simulink model "A1_MIM0_DigiTwin_4cm_JG_BM_2017b"  (R2017b)
settings: Solver=VariableStepAuto  StartTime=0.0  StopTime=tsim  RelTol=1e-3
InitFcn:
  | tsim=1000
  | sg=1;
  | Ts=500 %500% deseado 890-->Ts modelo
  | wn=5.8335/Ts; %2ord
  | wp=4/Ts; %np=1.5; 1ord
  | wt1=8*wn
  | wt=3.5*wn
  | wt3=3.49*wn
  | nf=2.5; %[1.2 1.5 1.75 2 2.5]
  | %Tfp=1/(np*wp)
  | Tf= 1/(nf*wn) % f del filtro;
  | nf3=5
  | Tf3= 1/(nf3*wn)
  | Rpc=0.09 % cold side resistor
  | Rph= 0.6 % hot side resistor
  | Tamb=273.15+15 % ambiental temp
  | Tin=273.15+15 % initial temp of mass
  | %TinA= 284.9405 % internal air Inicial temp
  | %TinAis=  294.0300 % initial Temp Mass insolat
  | %Tp1=283  %ideal temp of  peltier cells
  | %Tp2=Tp1
  | 
  | %Peltier Cells parameter
  | Th=323 % [K]
  | TinH=298
  | TinC=298 %
  | dTmax=75 % 70.5 [K]
  | Vmax= 16.4 % 13.9 [v]
  | Imax= 6.4 % 4  [A]
  | Rth= (dTmax/(Vmax*Imax))*(2*Th/(Th-dTmax)) % Termal Res [K/W]
  | am= Vmax/ Th %  0.054 Seebeck Coef []
  | ReC=Vmax*(Th-dTmax)/(Th*Imax) %range [1.6 1.96 2.5]
  | %Re= 2.3 %2.65   [2.6584  2.9592 3.26]  at 300 K
  | Mc=0.0135; %0.0045  Cool mass [kg]
  | Mh=0.0135; %0.0045
  | Cesp=1262  %1262.2 345
  | %TinL=300
  | %CespL=100 %45
  | %Mload=100%100-0.065 0.001
  | %Rload=1%5.5
  | 
  | 
  | % --Copper & aluminum plate
  | Da= 8960; %2700 [Kg/m^3] density
  | Qs= 390; %970 Specific heat [J/(Kg*K)]
  | Thi =0.00508; % 0.0033 Thickness [m]
  | L = 0.04; %0.03 length [m]
  | L1=0.035;
  | W=0.04; % 0.03 width  [m]
  | W1=0.01; W2=0.03;  W3=0.015;
  | Va= L*W*Thi % 2,97 E-6 [m^3] Dif of Volume
  | M=Da*Va % 0.00801 [kg]  % Al Dif of Mass
  | 
  | %--- Air Properties
  | Thi_air=0.015 % Thickness of air
  | Dair=1.29 % [Kg/m^3] density
  | Vair= L*W*Thi_air % E-6 [m^3] Dif of Volume
  | Mair=Dair*Vair %  [kg]  % Al Dif of Mass
  | 
  | % thermal conductivity [W/(m*K)]
  | ... (+57 lines)
undefined symbols (not defined in the file or in its folder): TinA, TinAis, ymax, ymin
libraries: fl_lib x233, nesl_utility x61, simulink x6, ee_lib x4
(part 2 of 2)

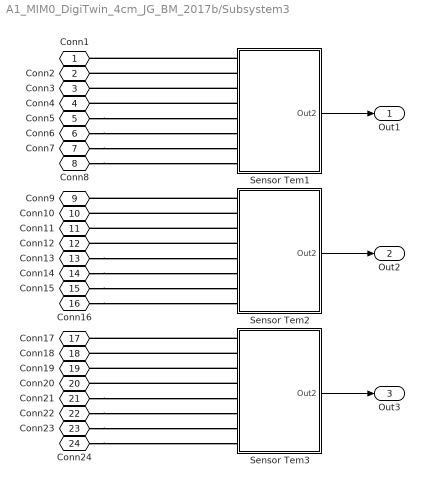
== system A1_MIM0_DigiTwin_4cm_JG_BM_2017b/Subsystem3 ==
  Sensor Tem1 : Subsystem
  Sensor Tem2 : Subsystem
  Sensor Tem3 : Subsystem
  Conn1 : PMIOPort  Side=Left
  Conn2 : PMIOPort  Port=2  Side=Left
  Conn3 : PMIOPort  Port=3  Side=Left
  Conn4 : PMIOPort  Port=4  Side=Left
  Conn5 : PMIOPort  Port=5  Side=Left
  Conn6 : PMIOPort  Port=6  Side=Left
  Conn7 : PMIOPort  Port=7  Side=Left
  Conn8 : PMIOPort  Port=8  Side=Left
  Conn9 : PMIOPort  Port=9  Side=Left
  Conn10 : PMIOPort  Port=10  Side=Left
  Conn11 : PMIOPort  Port=11  Side=Left
  Conn12 : PMIOPort  Port=12  Side=Left
  Conn13 : PMIOPort  Port=13  Side=Left
  Conn14 : PMIOPort  Port=14  Side=Left
  Conn15 : PMIOPort  Port=15  Side=Left
  Conn16 : PMIOPort  Port=16  Side=Left
  Conn17 : PMIOPort  Port=17  Side=Left
  Conn18 : PMIOPort  Port=18  Side=Left
  Conn19 : PMIOPort  Port=19  Side=Left
  Conn20 : PMIOPort  Port=20  Side=Left
  Conn21 : PMIOPort  Port=21  Side=Left
  Conn22 : PMIOPort  Port=22  Side=Left
  Conn23 : PMIOPort  Port=23  Side=Left
  Conn24 : PMIOPort  Port=24  Side=Left
  Out1 : Outport  VectorParamsAs1DForOutWhenUnconnected=off
  Out2 : Outport  Port=2  VectorParamsAs1DForOutWhenUnconnected=off
  Out3 : Outport  Port=3  VectorParamsAs1DForOutWhenUnconnected=off
  wires:
  Sensor Tem1/1(Out2) -> Out1/1
  Sensor Tem2/1(Out2) -> Out2/1
  Sensor Tem3/1(Out2) -> Out3/1
  connections:
  Sensor Tem1/LConn3 -- Conn3/RConn1
  Conn6/RConn1 -- Sensor Tem1/LConn6
  Conn7/RConn1 -- Sensor Tem1/LConn7
  Conn8/RConn1 -- Sensor Tem1/LConn8
  Sensor Tem1/LConn2 -- Conn2/RConn1
  Sensor Tem1/LConn4 -- Conn4/RConn1
  Conn5/RConn1 -- Sensor Tem1/LConn5
  Sensor Tem1/LConn1 -- Conn1/RConn1
  Conn13/RConn1 -- Sensor Tem2/LConn5
  Sensor Tem2/LConn4 -- Conn12/RConn1
  Conn16/RConn1 -- Sensor Tem2/LConn8
  Conn15/RConn1 -- Sensor Tem2/LConn7
  Sensor Tem2/LConn3 -- Conn11/RConn1
  Conn14/RConn1 -- Sensor Tem2/LConn6
  Sensor Tem2/LConn2 -- Conn10/RConn1
  Sensor Tem2/LConn1 -- Conn9/RConn1
  Conn21/RConn1 -- Sensor Tem3/LConn5
  Sensor Tem3/LConn4 -- Conn20/RConn1
  Conn24/RConn1 -- Sensor Tem3/LConn8
  Conn23/RConn1 -- Sensor Tem3/LConn7
  Conn22/RConn1 -- Sensor Tem3/LConn6
  Sensor Tem3/LConn3 -- Conn19/RConn1
  Sensor Tem3/LConn2 -- Conn18/RConn1
  Sensor Tem3/LConn1 -- Conn17/RConn1

== system A1_MIM0_DigiTwin_4cm_JG_BM_2017b/Subsystem4 ==
  PS-Simulink Converter1 : nesl_utility/PS-Simulink Converter  PhysicalDomain=network_engine_domain  SubClassName=ps_output  LeftPortType=input  RightPortType=output  PseudoPeriodic=off  Frequencies=[]  VectorFormat=1-D array  Unit=1  AffineConversion=off
  Temperature Sensor2 : fl_lib/Thermal/Thermal Sensors/Temperature Sensor
  Thermal Reference1 : fl_lib/Thermal/Thermal Elements/Thermal Reference
  Conn1 : PMIOPort  Side=Left
  Out1 : Outport  VectorParamsAs1DForOutWhenUnconnected=off
  wires:
  PS-Simulink Converter1/1 -> Out1/1
  connections:
  Thermal Reference1/LConn1 -- Temperature Sensor2/RConn1
  Temperature Sensor2/LConn1 -- Conn1/RConn1
  Temperature Sensor2/RConn2 -- PS-Simulink Converter1/LConn1

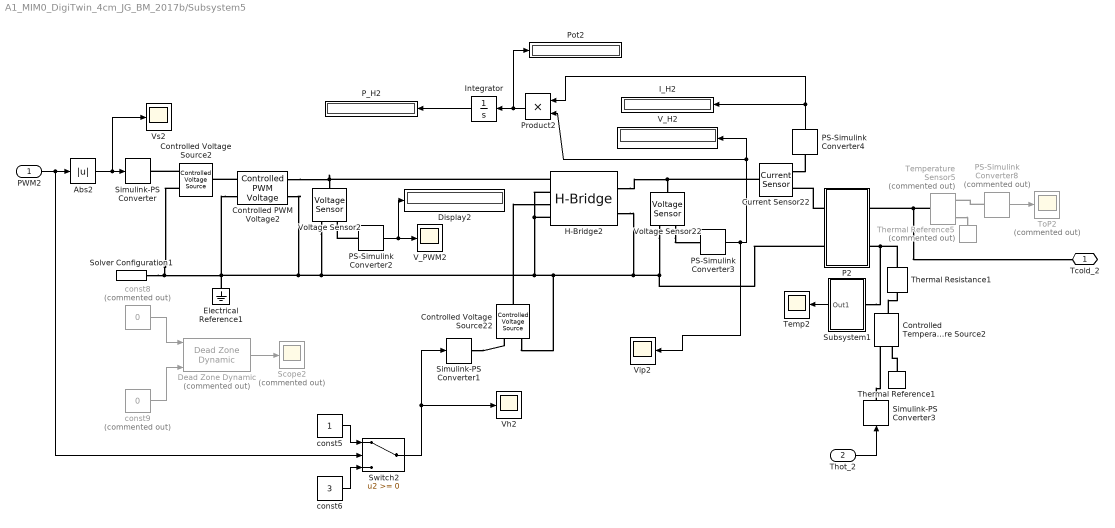
== system A1_MIM0_DigiTwin_4cm_JG_BM_2017b/Subsystem5 ==
  PWM2 : Inport
  Thot_2 : Inport  Port=2
  Abs2 : Abs
  Controlled Temperature Source2 : fl_lib/Thermal/Thermal Sources/Controlled Temperature Source
  Controlled PWM Voltage2 : ee_lib/Integrated Circuits/Controlled PWM Voltage  F=4000 Hz  TD=0 s  pulse_width_offset=0 s  pulse_min=0 s  pwm_or_av=2  event_type=1  sample_time=1e-6 s  Vmin=0 V  Vmax=5 V  Vm=5 V  u_min=0  u_max=1
  Controlled Voltage Source2 : fl_lib/Electrical/Electrical Sources/Controlled Voltage Source
  Controlled Voltage Source22 : fl_lib/Electrical/Electrical Sources/Controlled Voltage Source
  Current Sensor22 : fl_lib/Electrical/Electrical Sensors/Current Sensor
  Dead Zone Dynamic : simulink/Discontinuities/Dead Zone Dynamic  Commented=on
  Display2 : Display
  Electrical Reference1 : fl_lib/Electrical/Electrical Elements/Electrical Reference
  H-Bridge2 : ee_lib/Semiconductors & Converters/Converters/H-Bridge  supply_ports=ee.enum.supply_ports.hidesupply  pwm_or_av=2  regenerative_braking_mode=2  discontinuous=0  freewheeling_mode=1  Rload=10 Ohm  Lload=1e-5 H  F=10 kHz  Venable=2.5 V  Vmax=5.0 V  Vreverse=2.5 V  Vbrake=2.5 V  Vm=12 V  Ron=0.1 Ohm  Don=0.05 Ohm  Goff=1e-6 S  Tmeas=298.15 K  Ron2=0.1 Ohm  Don2=0.05 Ohm  Tmeas2=398.15 K  thermal_mass=100 J/K  initial_temperature=298.15 K
  I_H2 : Display
  Integrator : Integrator
  P2 : Subsystem
  PS-Simulink Converter2 : nesl_utility/PS-Simulink Converter  PhysicalDomain=network_engine_domain  SubClassName=ps_output  LeftPortType=input  RightPortType=output  PseudoPeriodic=off  Frequencies=[]  VectorFormat=1-D array  Unit=1  AffineConversion=off
  PS-Simulink Converter3 : nesl_utility/PS-Simulink Converter  PhysicalDomain=network_engine_domain  SubClassName=ps_output  LeftPortType=input  RightPortType=output  PseudoPeriodic=off  Frequencies=[]  VectorFormat=1-D array  Unit=1  AffineConversion=off
  PS-Simulink Converter4 : nesl_utility/PS-Simulink Converter  PhysicalDomain=network_engine_domain  SubClassName=ps_output  LeftPortType=input  RightPortType=output  PseudoPeriodic=off  Frequencies=[]  VectorFormat=1-D array  Unit=1  AffineConversion=off
  PS-Simulink Converter8 : nesl_utility/PS-Simulink Converter  Commented=on  PhysicalDomain=network_engine_domain  SubClassName=ps_output  LeftPortType=input  RightPortType=output  PseudoPeriodic=off  Frequencies=[]  VectorFormat=1-D array  Unit=1  AffineConversion=off
  P_H2 : Display
  Pot2 : Display
  Product2 : Product  RndMeth=Zero
  Scope2 : Scope  Commented=on
  Simulink-PS Converter : nesl_utility/Simulink-PS Converter  PhysicalDomain=network_engine_domain  SubClassName=ps_input  LeftPortType=input  RightPortType=output  PseudoPeriodic=off  Frequencies=[]  NoiseDistribution=none  NoiseParameters=[]  Unit=1  AffineConversion=off  FilteringAndDerivatives=provide  SimscapeFilterOrder=1  InputFilterTimeConstant=0.001  UdotUserProvided=0
  Simulink-PS Converter1 : nesl_utility/Simulink-PS Converter  PhysicalDomain=network_engine_domain  SubClassName=ps_input  LeftPortType=input  RightPortType=output  PseudoPeriodic=off  Frequencies=[]  NoiseDistribution=none  NoiseParameters=[]  Unit=1  AffineConversion=off  FilteringAndDerivatives=provide  SimscapeFilterOrder=1  InputFilterTimeConstant=0.001  UdotUserProvided=0
  Simulink-PS Converter3 : nesl_utility/Simulink-PS Converter  PhysicalDomain=network_engine_domain  SubClassName=ps_input  LeftPortType=input  RightPortType=output  PseudoPeriodic=off  Frequencies=[]  NoiseDistribution=none  NoiseParameters=[]  Unit=1  AffineConversion=off  FilteringAndDerivatives=provide  SimscapeFilterOrder=1  InputFilterTimeConstant=0.001  UdotUserProvided=0
  Solver Configuration1 : nesl_utility/Solver Configuration  PhysicalDomain=network_engine_domain  SubClassName=solver  LeftPortType=input  RightPortType=generic  Tones=[]  Harmonics=[]  SimulateNoise=off  Profile=off  UseLocalSampling=off  EnableSwitchedLinearOptims=on  FrequencyDomain=off  UseCCode=off  RelTol=0.001  AbsTol=1e-06  MinStep=1e-09  ToWorkspace=off  RevertToSquareIcSolve=off  NumHomotopyIterations=100  PhasorMode=off  PhasorModeNumHarmonics=1  ConsistencySolver=NEWTON_FTOL  IndexReductionMethod=DerivativeReplacement  DoDC=off  ResidualTolerance=1e-09  ConsistencyTolSource=GLOBAL  ConsistencyAbsTol=0.001  ConsistencyRelTol=0.001  ConsistencyTolFactor=0.001  UseLocalSolver=off  LocalSolverChoice=NE_BACKWARD_EULER_ADVANCER  ResolveIndetEquations=on  FunctionEvalNumThread=1  LocalSolverSampleTime=0.001  DoFixedCost=off  MaxNonlinIter=3  MaxModeIter=2  ComputeImpulses=off  ImpulseIterations=2  LinearAlgebra=Sparse  LinearAlgebraNumThread=0  EquationFormulation=NE_TIME_EF  DelaysMemoryBudget=1024  AutomaticFiltering=on  FilteringTimeConstant=0.001  PartitionStorageMethod=AS_NEEDED  PartitionMemoryBudget=1024  PartitionMethod=FAST
  Subsystem1 : Subsystem
  Switch2 : Switch
  Temp2 : Scope
  Temperature Sensor5 : fl_lib/Thermal/Thermal Sensors/Temperature Sensor  Commented=on
  Thermal Reference1 : fl_lib/Thermal/Thermal Elements/Thermal Reference
  Thermal Reference5 : fl_lib/Thermal/Thermal Elements/Thermal Reference  Commented=on
  Thermal Resistance1 : fl_lib/Thermal/Thermal Elements/Thermal Resistance  resistance=Rph K/W  T_specify=off  T_priority=None  T=0 K  T_nominal_specify=off  T_nominal_unit=K  T_nominal_value=1  Q_specify=off  Q_priority=None  Q=0 W  Q_nominal_specify=off  Q_nominal_unit=W  Q_nominal_value=1
  ToP2 : Scope  Commented=on
  V_H2 : Display
  V_PWM2 : Scope
  Vh2 : Scope
  Vip2 : Scope
  Voltage Sensor2 : fl_lib/Electrical/Electrical Sensors/Voltage Sensor
  Voltage Sensor22 : fl_lib/Electrical/Electrical Sensors/Voltage Sensor
  Vs2 : Scope
  const5 : Constant
  const6 : Constant  Value=3
  const8 : Constant  Commented=on  Value=0
  const9 : Constant  Commented=on  Value=0
  Tcold_2 : PMIOPort  Side=Right
  wires:
  const8/1 -> Dead Zone Dynamic/1
  Dead Zone Dynamic/1 -> Scope2/1
  const9/1 -> Dead Zone Dynamic/3
  Product2/1 -> Integrator/1, Pot2/1
  PS-Simulink Converter3/1 -> V_H2/1, Product2/2, Vip2/1
  PS-Simulink Converter4/1 -> I_H2/1, Product2/1
  Integrator/1 -> P_H2/1
  Abs2/1 -> Simulink-PS Converter/1, Vs2/1
  const6/1 -> Switch2/3
  PWM2/1 -> Abs2/1, Switch2/2
  const5/1 -> Switch2/1
  Thot_2/1 -> Simulink-PS Converter3/1
  Subsystem1/1(Out1) -> Temp2/1
  PS-Simulink Converter2/1 -> V_PWM2/1, Display2/1
  PS-Simulink Converter8/1 -> ToP2/1
  Switch2/1 -> Vh2/1, Simulink-PS Converter1/1
  connections:
  Controlled PWM Voltage2/LConn2 -- Controlled PWM Voltage2/RConn2 -- Voltage Sensor2/RConn2 -- H-Bridge2/RConn2 -- Voltage Sensor22/RConn2 -- P2/LConn2 -- Controlled Voltage Source22/RConn2 -- H-Bridge2/LConn2 -- H-Bridge2/LConn4 -- Solver Configuration1/RConn1 -- Controlled Voltage Source2/RConn2 -- Electrical Reference1/LConn1
  Controlled Temperature Source2/LConn1 -- Thermal Resistance1/LConn1
  Thermal Reference1/LConn1 -- Controlled Temperature Source2/RConn2
  Simulink-PS Converter3/RConn1 -- Controlled Temperature Source2/RConn1
  P2/RConn2 -- Subsystem1/LConn1 -- Thermal Resistance1/RConn1
  Current Sensor22/RConn1 -- PS-Simulink Converter4/LConn1
  Voltage Sensor22/LConn1 -- Current Sensor22/LConn1 -- H-Bridge2/RConn1
  PS-Simulink Converter2/LConn1 -- Voltage Sensor2/RConn1
  P2/RConn1 -- Tcold_2/RConn1 -- Temperature Sensor5/LConn1
  Controlled Voltage Source2/RConn1 -- Simulink-PS Converter/RConn1
  Voltage Sensor2/LConn1 -- H-Bridge2/LConn1 -- Controlled PWM Voltage2/RConn1
  Voltage Sensor22/RConn1 -- PS-Simulink Converter3/LConn1
  PS-Simulink Converter8/LConn1 -- Temperature Sensor5/RConn2
  Controlled Voltage Source22/LConn1 -- H-Bridge2/LConn3
  Controlled PWM Voltage2/LConn1 -- Controlled Voltage Source2/LConn1
  P2/LConn1 -- Current Sensor22/RConn2
  Simulink-PS Converter1/RConn1 -- Controlled Voltage Source22/RConn1
  Temperature Sensor5/RConn1 -- Thermal Reference5/LConn1

== system A1_MIM0_DigiTwin_4cm_JG_BM_2017b/Subsystem6 ==
  PS-Simulink Converter1 : nesl_utility/PS-Simulink Converter  PhysicalDomain=network_engine_domain  SubClassName=ps_output  LeftPortType=input  RightPortType=output  PseudoPeriodic=off  Frequencies=[]  VectorFormat=1-D array  Unit=1  AffineConversion=off
  Temperature Sensor2 : fl_lib/Thermal/Thermal Sensors/Temperature Sensor
  Thermal Reference1 : fl_lib/Thermal/Thermal Elements/Thermal Reference
  Conn1 : PMIOPort  Side=Left
  Out1 : Outport  VectorParamsAs1DForOutWhenUnconnected=off
  wires:
  PS-Simulink Converter1/1 -> Out1/1
  connections:
  Temperature Sensor2/RConn2 -- PS-Simulink Converter1/LConn1
  Temperature Sensor2/LConn1 -- Conn1/RConn1
  Thermal Reference1/LConn1 -- Temperature Sensor2/RConn1

== system A1_MIM0_DigiTwin_4cm_JG_BM_2017b/Subsystem7 ==
  PS-Simulink Converter1 : nesl_utility/PS-Simulink Converter  PhysicalDomain=network_engine_domain  SubClassName=ps_output  LeftPortType=input  RightPortType=output  PseudoPeriodic=off  Frequencies=[]  VectorFormat=1-D array  Unit=1  AffineConversion=off
  Temperature Sensor2 : fl_lib/Thermal/Thermal Sensors/Temperature Sensor
  Thermal Reference4 : fl_lib/Thermal/Thermal Elements/Thermal Reference
  Conn1 : PMIOPort  Side=Left
  Out1 : Outport  VectorParamsAs1DForOutWhenUnconnected=off
  wires:
  PS-Simulink Converter1/1 -> Out1/1
  connections:
  Thermal Reference4/LConn1 -- Temperature Sensor2/RConn1
  PS-Simulink Converter1/LConn1 -- Temperature Sensor2/RConn2
  Temperature Sensor2/LConn1 -- Conn1/RConn1

== system A1_MIM0_DigiTwin_4cm_JG_BM_2017b/Ts_98%1 ==
  note: Subsystem
  note: Subsystem1
  In1 : Inport
  Constant1 : Constant  Commented=on  Value=ymax
  Constant4 : Constant  Value=298
  Constant5 : Constant  Commented=on  Value=ymin
  Manual Switch : ManualSwitch  Commented=on  CurrentSetting=0
  MpSinF : TransferFcn  Numerator=1  Denominator=[(1/wp) 1]
  MrF1ord1 : TransferFcn  Numerator=[wn^2*Tf wn^2]  Denominator=[1 2*wn*sg wn^2 ]
  MrWn1 : TransferFcn  Numerator=[wn^2]  Denominator=[1 2*wn*sg wn^2 ]
  Product : Product
  Product1 : Product
  Repeating Sequence Stair1 : simulink/Sources/Repeating Sequence Stair  OutValues=[ 0 1 0 ]'  tsamp=2000  OutMin=[]  OutMax=[]  OutDataTypeStr=float('double')  OutputDataTypeScalingMode=Specify via dialog  OutDataType=float('double')  ConRadixGroup=Best Precision: Vector-wise  OutScaling=2^-12
  Repeating Sequence Stair2 : simulink/Sources/Repeating Sequence Stair  OutValues=[ 1 0 1 ]'  tsamp=2000  OutMin=[]  OutMax=[]  OutDataTypeStr=float('double')  OutputDataTypeScalingMode=Specify via dialog  OutDataType=float('double')  ConRadixGroup=Best Precision: Vector-wise  OutScaling=2^-12
  Subtract : Sum  Inputs=+-
  Subtract1 : Sum
  Yab : Constant  Value=-10.2170e+000
  Ymax : Constant  Value=44.2455e+000
  Ymin : Constant  Value=-11.3285e+000
  yar : Constant  Value=43.3605e+000
  Peltier : Outport  VectorParamsAs1DForOutWhenUnconnected=off
  Out2 : Outport  Port=2  VectorParamsAs1DForOutWhenUnconnected=off
  Out3 : Outport  Port=3  VectorParamsAs1DForOutWhenUnconnected=off
  Ms : Outport  Port=4  VectorParamsAs1DForOutWhenUnconnected=off
  MsFp : Outport  Port=5  VectorParamsAs1DForOutWhenUnconnected=off
  Mp : Outport  Port=6  VectorParamsAs1DForOutWhenUnconnected=off
  wires:
  yar/1 -> Out2/1
  Yab/1 -> Out3/1
  Constant4/1 -> Subtract/2
  Subtract/1 -> Peltier/1
  In1/1 -> Subtract/1
  Product1/1 -> Subtract1/2
  Ymax/1 -> Product/1
  Product/1 -> Subtract1/1
  Repeating Sequence Stair2/1 -> Product/2
  Repeating Sequence Stair1/1 -> Product1/1
  Ymin/1 -> Product1/2
  MrWn1/1 -> Ms/1
  MrF1ord1/1 -> MsFp/1
  MpSinF/1 -> Mp/1
  Subtract1/1 -> MrWn1/1, MpSinF/1, MrF1ord1/1

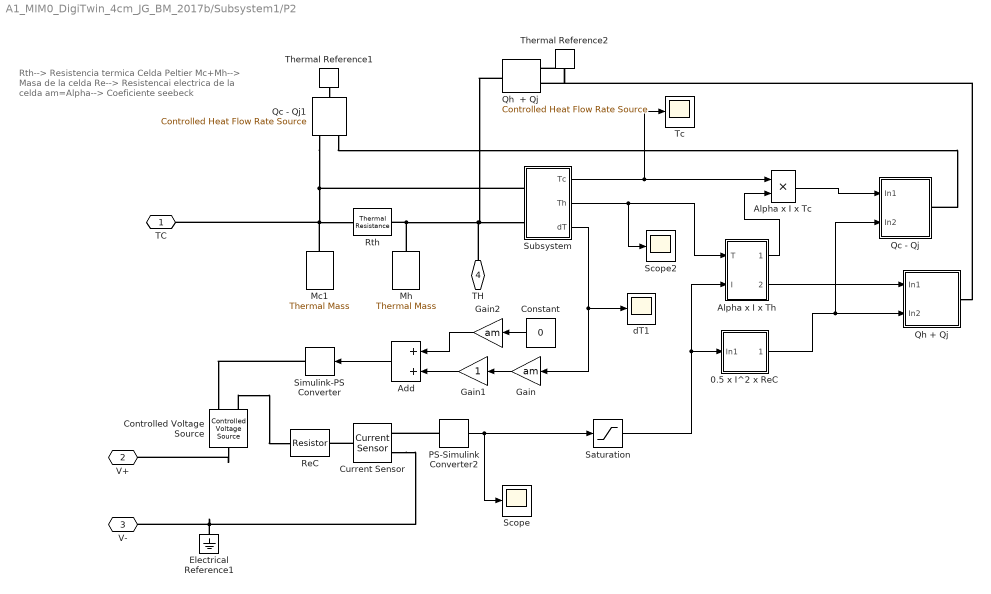
== system A1_MIM0_DigiTwin_4cm_JG_BM_2017b/Subsystem1/P2 ==
  note: Rth-->                  Resistencia termica Celda Peltier
      | Mc+Mh-->            Masa de la celda
      | Re-->                  Resistencai electrica de la celda
      | am=Alpha-->       Coeficiente seebeck
  0.5 x I^2 x ReC : Subsystem
  Add : Sum
  Alpha x I x Tc : Product
  Alpha x I x Th : Subsystem
  Constant : Constant  Value=0
  Controlled Voltage Source : fl_lib/Electrical/Electrical Sources/Controlled Voltage Source
  Current Sensor : fl_lib/Electrical/Electrical Sensors/Current Sensor
  Electrical Reference1 : fl_lib/Electrical/Electrical Elements/Electrical Reference
  Gain : Gain  Gain=am
  Gain1 : Gain
  Gain2 : Gain  Gain=am
  Mc1 : fl_lib/Thermal/Thermal Elements/Thermal Mass  mass=Mc kg  sp_heat=Cesp J/kg/K  num_ports=foundation.enum.numPorts2.one  T_specify=on  T_priority=High  T=TinC K  T_nominal_specify=off  T_nominal_unit=K  T_nominal_value=1  Q_specify=off  Q_priority=None  Q=0 W  Q_nominal_specify=off  Q_nominal_unit=W  Q_nominal_value=1
  Mh : fl_lib/Thermal/Thermal Elements/Thermal Mass  mass=Mh kg  sp_heat=Cesp J/kg/K  num_ports=foundation.enum.numPorts2.one  T_specify=on  T_priority=High  T=TinH K  T_nominal_specify=off  T_nominal_unit=K  T_nominal_value=1  Q_specify=off  Q_priority=None  Q=0 W  Q_nominal_specify=off  Q_nominal_unit=W  Q_nominal_value=1
  PS-Simulink Converter2 : nesl_utility/PS-Simulink Converter  PhysicalDomain=network_engine_domain  SubClassName=ps_output  LeftPortType=input  RightPortType=output  PseudoPeriodic=off  Frequencies=[]  VectorFormat=1-D array  Unit=1  AffineConversion=off
  "Qc - Qj " : Subsystem
  "Qc - Qj1 " : fl_lib/Thermal/Thermal Sources/Controlled Heat Flow Rate Source
  Qh  + Qj : fl_lib/Thermal/Thermal Sources/Controlled Heat Flow Rate Source
  "Qh + Qj " : Subsystem
  ReC : fl_lib/Electrical/Electrical Elements/Resistor  R=ReC Ohm  i_specify=off  i_priority=None  i=0 A  i_nominal_specify=off  i_nominal_unit=A  i_nominal_value=1  v_specify=off  v_priority=None  v=0 V  v_nominal_specify=off  v_nominal_unit=V  v_nominal_value=1
  Rth : fl_lib/Thermal/Thermal Elements/Thermal Resistance  resistance=Rth K/W  T_specify=off  T_priority=None  T=0 K  T_nominal_specify=off  T_nominal_unit=K  T_nominal_value=1  Q_specify=off  Q_priority=None  Q=0 W  Q_nominal_specify=off  Q_nominal_unit=W  Q_nominal_value=1
  Saturation : Saturate  UpperLimit=inf  LowerLimit=-inf
  Scope : Scope
  Scope2 : Scope
  Simulink-PS Converter : nesl_utility/Simulink-PS Converter  PhysicalDomain=network_engine_domain  SubClassName=ps_input  LeftPortType=input  RightPortType=output  PseudoPeriodic=off  Frequencies=[]  NoiseDistribution=none  NoiseParameters=[]  Unit=1  AffineConversion=off  FilteringAndDerivatives=provide  SimscapeFilterOrder=1  InputFilterTimeConstant=0.001  UdotUserProvided=0
  Subsystem : Subsystem
  Tc : Scope
  Thermal Reference1 : fl_lib/Thermal/Thermal Elements/Thermal Reference
  Thermal Reference2 : fl_lib/Thermal/Thermal Elements/Thermal Reference
  dT1 : Scope
  TC : PMIOPort  Side=Right
  V+ : PMIOPort  Port=2  Side=Left
  V- : PMIOPort  Port=3  Side=Left
  TH : PMIOPort  Port=4  Side=Right
  wires:
  PS-Simulink Converter2/1 -> Scope/1, Saturation/1
  0.5 x I^2 x ReC/1(Out1) -> "Qc - Qj "/2(In2), "Qh + Qj "/2(In2)
  Subsystem/1(Tc) -> Tc/1, Alpha x I x Tc/1
  Alpha x I x Th/1(Out1) -> Alpha x I x Tc/2
  Alpha x I x Tc/1 -> "Qc - Qj "/1(In1)
  Alpha x I x Th/2(Out2) -> "Qh + Qj "/1(In1)
  Subsystem/2(Th) -> Scope2/1, Alpha x I x Th/1(T)
  Saturation/1 -> Alpha x I x Th/2(I), 0.5 x I^2 x ReC/1(In1)
  Subsystem/3(dT) -> Gain/1, dT1/1
  Gain/1 -> Gain1/1
  Gain1/1 -> Add/2
  Constant/1 -> Gain2/1
  Add/1 -> Simulink-PS Converter/1
  Gain2/1 -> Add/1
  connections:
  Current Sensor/LConn1 -- ReC/RConn1
  Thermal Reference1/LConn1 -- "Qc - Qj1 "/LConn1
  Thermal Reference2/LConn1 -- Qh  + Qj/RConn2
  Mh/LConn1 -- Rth/RConn1 -- Qh  + Qj/LConn1 -- Subsystem/LConn2 -- TH/RConn1
  Simulink-PS Converter/RConn1 -- Controlled Voltage Source/RConn1
  Controlled Voltage Source/RConn2 -- ReC/LConn1
  PS-Simulink Converter2/LConn1 -- Current Sensor/RConn1
  Controlled Voltage Source/LConn1 -- V+/RConn1
  Current Sensor/RConn2 -- V-/RConn1 -- Electrical Reference1/LConn1
  "Qc - Qj1 "/RConn1 -- "Qc - Qj "/RConn1
  "Qh + Qj "/RConn1 -- Qh  + Qj/RConn1
  "Qc - Qj1 "/RConn2 -- Subsystem/LConn1 -- Mc1/LConn1 -- TC/RConn1 -- Rth/LConn1

== system A1_MIM0_DigiTwin_4cm_JG_BM_2017b/Subsystem1/Subsystem1 ==
  PS-Simulink Converter7 : nesl_utility/PS-Simulink Converter  PhysicalDomain=network_engine_domain  SubClassName=ps_output  LeftPortType=input  RightPortType=output  PseudoPeriodic=off  Frequencies=[]  VectorFormat=1-D array  Unit=1  AffineConversion=off
  Temperature Sensor1 : fl_lib/Thermal/Thermal Sensors/Temperature Sensor
  Thermal Reference2 : fl_lib/Thermal/Thermal Elements/Thermal Reference
  Conn1 : PMIOPort  Side=Left
  Out1 : Outport  VectorParamsAs1DForOutWhenUnconnected=off
  wires:
  PS-Simulink Converter7/1 -> Out1/1
  connections:
  Thermal Reference2/LConn1 -- Temperature Sensor1/RConn1
  PS-Simulink Converter7/LConn1 -- Temperature Sensor1/RConn2
  Temperature Sensor1/LConn1 -- Conn1/RConn1

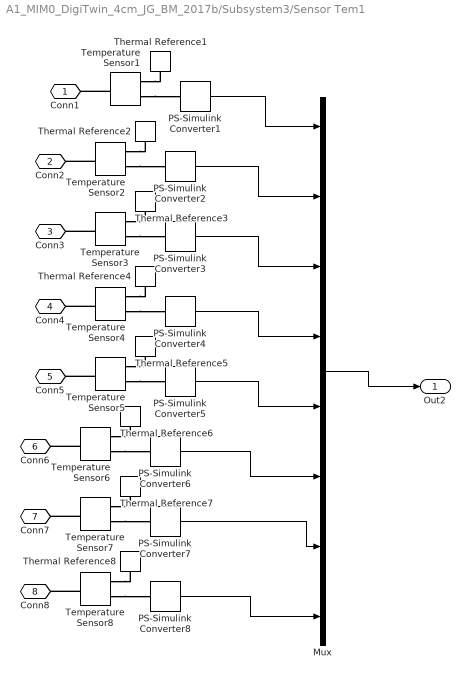
== system A1_MIM0_DigiTwin_4cm_JG_BM_2017b/Subsystem3/Sensor Tem1 ==
  Mux : Mux  Inputs=8
  PS-Simulink Converter{1..8} (8 alike) : nesl_utility/PS-Simulink Converter  PhysicalDomain=network_engine_domain  SubClassName=ps_output  LeftPortType=input  RightPortType=output  PseudoPeriodic=off  Frequencies=[]  VectorFormat=1-D array  Unit=1  AffineConversion=off
  Temperature Sensor{1..8} (8 alike) : fl_lib/Thermal/Thermal Sensors/Temperature Sensor
  Thermal Reference{1..8} (8 alike) : fl_lib/Thermal/Thermal Elements/Thermal Reference
  Conn1 : PMIOPort  Side=Left
  Conn2 : PMIOPort  Port=2  Side=Left
  Conn3 : PMIOPort  Port=3  Side=Left
  Conn4 : PMIOPort  Port=4  Side=Left
  Conn5 : PMIOPort  Port=5  Side=Left
  Conn6 : PMIOPort  Port=6  Side=Left
  Conn7 : PMIOPort  Port=7  Side=Left
  Conn8 : PMIOPort  Port=8  Side=Left
  Out2 : Outport  VectorParamsAs1DForOutWhenUnconnected=off
  wires:
  PS-Simulink Converter5/1 -> Mux/5
  PS-Simulink Converter7/1 -> Mux/7
  PS-Simulink Converter8/1 -> Mux/8
  PS-Simulink Converter6/1 -> Mux/6
  PS-Simulink Converter4/1 -> Mux/4
  PS-Simulink Converter3/1 -> Mux/3
  PS-Simulink Converter1/1 -> Mux/1
  PS-Simulink Converter2/1 -> Mux/2
  Mux/1 -> Out2/1
  connections:
  Temperature Sensor6/RConn2 -- PS-Simulink Converter6/LConn1
  Temperature Sensor5/RConn2 -- PS-Simulink Converter5/LConn1
  Temperature Sensor5/RConn1 -- Thermal Reference5/LConn1
  Temperature Sensor7/RConn2 -- PS-Simulink Converter7/LConn1
  Temperature Sensor6/RConn1 -- Thermal Reference6/LConn1
  Temperature Sensor5/LConn1 -- Conn5/RConn1
  Temperature Sensor6/LConn1 -- Conn6/RConn1
  Temperature Sensor7/LConn1 -- Conn7/RConn1
  Temperature Sensor7/RConn1 -- Thermal Reference7/LConn1
  Temperature Sensor8/RConn1 -- Thermal Reference8/LConn1
  Temperature Sensor8/LConn1 -- Conn8/RConn1
  Temperature Sensor8/RConn2 -- PS-Simulink Converter8/LConn1
  Temperature Sensor4/RConn2 -- PS-Simulink Converter4/LConn1
  Temperature Sensor4/LConn1 -- Conn4/RConn1
  Temperature Sensor4/RConn1 -- Thermal Reference4/LConn1
  Temperature Sensor3/RConn1 -- Thermal Reference3/LConn1
  Temperature Sensor3/LConn1 -- Conn3/RConn1
  Temperature Sensor3/RConn2 -- PS-Simulink Converter3/LConn1
  Temperature Sensor2/RConn1 -- Thermal Reference2/LConn1
  Temperature Sensor2/RConn2 -- PS-Simulink Converter2/LConn1
  Temperature Sensor2/LConn1 -- Conn2/RConn1
  Temperature Sensor1/LConn1 -- Conn1/RConn1
  Temperature Sensor1/RConn2 -- PS-Simulink Converter1/LConn1
  Temperature Sensor1/RConn1 -- Thermal Reference1/LConn1

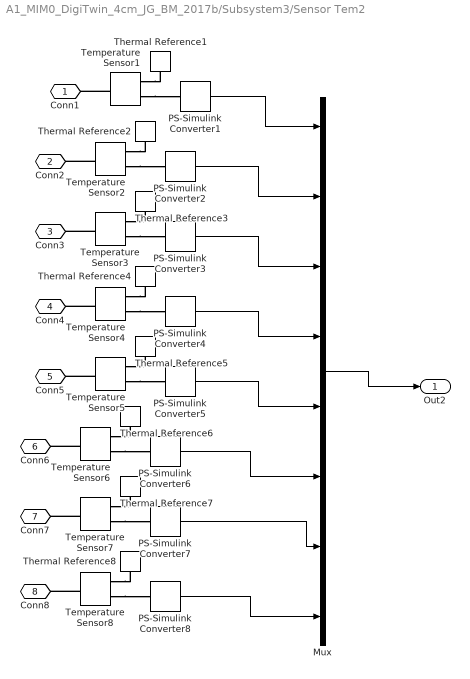
== system A1_MIM0_DigiTwin_4cm_JG_BM_2017b/Subsystem3/Sensor Tem2 ==
  Mux : Mux  Inputs=8
  PS-Simulink Converter{1..8} (8 alike) : nesl_utility/PS-Simulink Converter  PhysicalDomain=network_engine_domain  SubClassName=ps_output  LeftPortType=input  RightPortType=output  PseudoPeriodic=off  Frequencies=[]  VectorFormat=1-D array  Unit=1  AffineConversion=off
  Temperature Sensor{1..8} (8 alike) : fl_lib/Thermal/Thermal Sensors/Temperature Sensor
  Thermal Reference{1..8} (8 alike) : fl_lib/Thermal/Thermal Elements/Thermal Reference
  Conn1 : PMIOPort  Side=Left
  Conn2 : PMIOPort  Port=2  Side=Left
  Conn3 : PMIOPort  Port=3  Side=Left
  Conn4 : PMIOPort  Port=4  Side=Left
  Conn5 : PMIOPort  Port=5  Side=Left
  Conn6 : PMIOPort  Port=6  Side=Left
  Conn7 : PMIOPort  Port=7  Side=Left
  Conn8 : PMIOPort  Port=8  Side=Left
  Out2 : Outport  VectorParamsAs1DForOutWhenUnconnected=off
  wires:
  Mux/1 -> Out2/1
  PS-Simulink Converter2/1 -> Mux/2
  PS-Simulink Converter1/1 -> Mux/1
  PS-Simulink Converter3/1 -> Mux/3
  PS-Simulink Converter4/1 -> Mux/4
  PS-Simulink Converter6/1 -> Mux/6
  PS-Simulink Converter8/1 -> Mux/8
  PS-Simulink Converter7/1 -> Mux/7
  PS-Simulink Converter5/1 -> Mux/5
  connections:
  Temperature Sensor1/RConn1 -- Thermal Reference1/LConn1
  Temperature Sensor1/RConn2 -- PS-Simulink Converter1/LConn1
  Temperature Sensor1/LConn1 -- Conn1/RConn1
  Temperature Sensor2/LConn1 -- Conn2/RConn1
  Temperature Sensor2/RConn2 -- PS-Simulink Converter2/LConn1
  Temperature Sensor2/RConn1 -- Thermal Reference2/LConn1
  Temperature Sensor3/RConn2 -- PS-Simulink Converter3/LConn1
  Temperature Sensor3/LConn1 -- Conn3/RConn1
  Temperature Sensor3/RConn1 -- Thermal Reference3/LConn1
  Temperature Sensor4/RConn1 -- Thermal Reference4/LConn1
  Temperature Sensor4/LConn1 -- Conn4/RConn1
  Temperature Sensor4/RConn2 -- PS-Simulink Converter4/LConn1
  Temperature Sensor8/RConn2 -- PS-Simulink Converter8/LConn1
  Temperature Sensor8/LConn1 -- Conn8/RConn1
  Temperature Sensor8/RConn1 -- Thermal Reference8/LConn1
  Temperature Sensor7/RConn1 -- Thermal Reference7/LConn1
  Temperature Sensor7/LConn1 -- Conn7/RConn1
  Temperature Sensor6/LConn1 -- Conn6/RConn1
  Temperature Sensor5/LConn1 -- Conn5/RConn1
  Temperature Sensor6/RConn1 -- Thermal Reference6/LConn1
  Temperature Sensor7/RConn2 -- PS-Simulink Converter7/LConn1
  Temperature Sensor5/RConn1 -- Thermal Reference5/LConn1
  Temperature Sensor5/RConn2 -- PS-Simulink Converter5/LConn1
  Temperature Sensor6/RConn2 -- PS-Simulink Converter6/LConn1

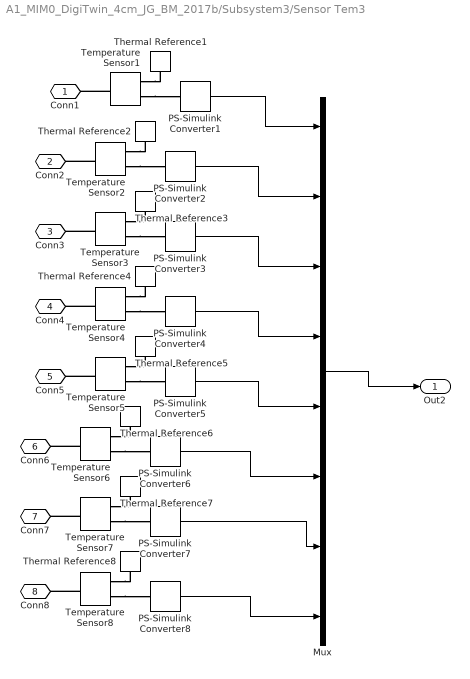
== system A1_MIM0_DigiTwin_4cm_JG_BM_2017b/Subsystem3/Sensor Tem3 ==
  Mux : Mux  Inputs=8
  PS-Simulink Converter{1..8} (8 alike) : nesl_utility/PS-Simulink Converter  PhysicalDomain=network_engine_domain  SubClassName=ps_output  LeftPortType=input  RightPortType=output  PseudoPeriodic=off  Frequencies=[]  VectorFormat=1-D array  Unit=1  AffineConversion=off
  Temperature Sensor{1..8} (8 alike) : fl_lib/Thermal/Thermal Sensors/Temperature Sensor
  Thermal Reference{1..8} (8 alike) : fl_lib/Thermal/Thermal Elements/Thermal Reference
  Conn1 : PMIOPort  Side=Left
  Conn2 : PMIOPort  Port=2  Side=Left
  Conn3 : PMIOPort  Port=3  Side=Left
  Conn4 : PMIOPort  Port=4  Side=Left
  Conn5 : PMIOPort  Port=5  Side=Left
  Conn6 : PMIOPort  Port=6  Side=Left
  Conn7 : PMIOPort  Port=7  Side=Left
  Conn8 : PMIOPort  Port=8  Side=Left
  Out2 : Outport  VectorParamsAs1DForOutWhenUnconnected=off
  wires:
  Mux/1 -> Out2/1
  PS-Simulink Converter2/1 -> Mux/2
  PS-Simulink Converter1/1 -> Mux/1
  PS-Simulink Converter3/1 -> Mux/3
  PS-Simulink Converter4/1 -> Mux/4
  PS-Simulink Converter6/1 -> Mux/6
  PS-Simulink Converter8/1 -> Mux/8
  PS-Simulink Converter7/1 -> Mux/7
  PS-Simulink Converter5/1 -> Mux/5
  connections:
  Temperature Sensor1/RConn1 -- Thermal Reference1/LConn1
  Temperature Sensor1/RConn2 -- PS-Simulink Converter1/LConn1
  Temperature Sensor1/LConn1 -- Conn1/RConn1
  Temperature Sensor2/LConn1 -- Conn2/RConn1
  Temperature Sensor2/RConn2 -- PS-Simulink Converter2/LConn1
  Temperature Sensor2/RConn1 -- Thermal Reference2/LConn1
  Temperature Sensor3/RConn2 -- PS-Simulink Converter3/LConn1
  Temperature Sensor3/LConn1 -- Conn3/RConn1
  Temperature Sensor3/RConn1 -- Thermal Reference3/LConn1
  Temperature Sensor4/RConn1 -- Thermal Reference4/LConn1
  Temperature Sensor4/LConn1 -- Conn4/RConn1
  Temperature Sensor4/RConn2 -- PS-Simulink Converter4/LConn1
  Temperature Sensor8/RConn2 -- PS-Simulink Converter8/LConn1
  Temperature Sensor8/LConn1 -- Conn8/RConn1
  Temperature Sensor8/RConn1 -- Thermal Reference8/LConn1
  Temperature Sensor7/RConn1 -- Thermal Reference7/LConn1
  Temperature Sensor7/LConn1 -- Conn7/RConn1
  Temperature Sensor6/LConn1 -- Conn6/RConn1
  Temperature Sensor5/LConn1 -- Conn5/RConn1
  Temperature Sensor6/RConn1 -- Thermal Reference6/LConn1
  Temperature Sensor7/RConn2 -- PS-Simulink Converter7/LConn1
  Temperature Sensor5/RConn1 -- Thermal Reference5/LConn1
  Temperature Sensor5/RConn2 -- PS-Simulink Converter5/LConn1
  Temperature Sensor6/RConn2 -- PS-Simulink Converter6/LConn1

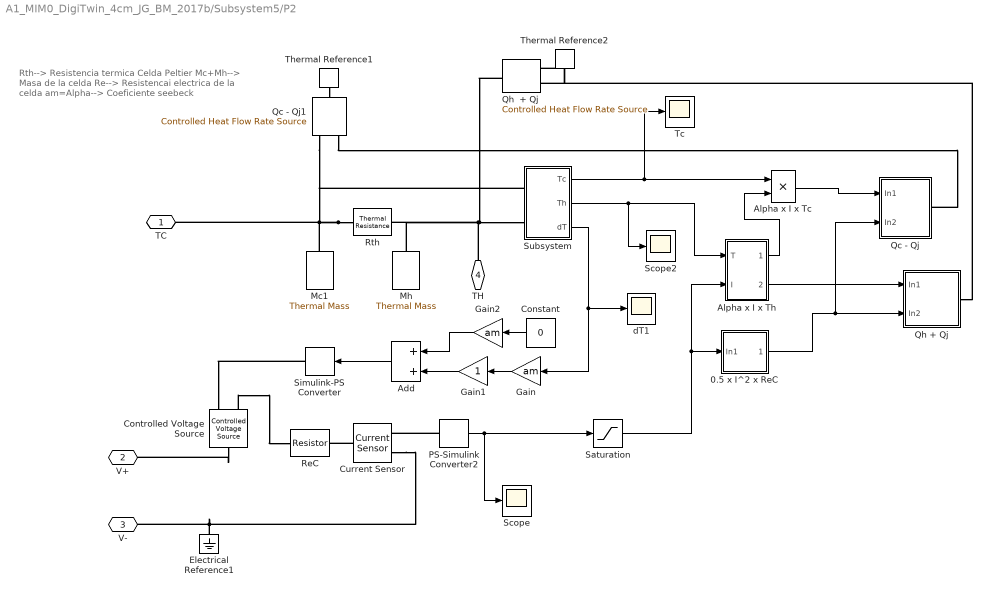
== system A1_MIM0_DigiTwin_4cm_JG_BM_2017b/Subsystem5/P2 ==
  note: Rth-->                  Resistencia termica Celda Peltier
      | Mc+Mh-->            Masa de la celda
      | Re-->                  Resistencai electrica de la celda
      | am=Alpha-->       Coeficiente seebeck
  0.5 x I^2 x ReC : Subsystem
  Add : Sum
  Alpha x I x Tc : Product
  Alpha x I x Th : Subsystem
  Constant : Constant  Value=0
  Controlled Voltage Source : fl_lib/Electrical/Electrical Sources/Controlled Voltage Source
  Current Sensor : fl_lib/Electrical/Electrical Sensors/Current Sensor
  Electrical Reference1 : fl_lib/Electrical/Electrical Elements/Electrical Reference
  Gain : Gain  Gain=am
  Gain1 : Gain
  Gain2 : Gain  Gain=am
  Mc1 : fl_lib/Thermal/Thermal Elements/Thermal Mass  mass=Mc kg  sp_heat=Cesp J/kg/K  num_ports=foundation.enum.numPorts2.one  T_specify=on  T_priority=High  T=TinC K  T_nominal_specify=off  T_nominal_unit=K  T_nominal_value=1  Q_specify=off  Q_priority=None  Q=0 W  Q_nominal_specify=off  Q_nominal_unit=W  Q_nominal_value=1
  Mh : fl_lib/Thermal/Thermal Elements/Thermal Mass  mass=Mh kg  sp_heat=Cesp J/kg/K  num_ports=foundation.enum.numPorts2.one  T_specify=on  T_priority=High  T=TinH K  T_nominal_specify=off  T_nominal_unit=K  T_nominal_value=1  Q_specify=off  Q_priority=None  Q=0 W  Q_nominal_specify=off  Q_nominal_unit=W  Q_nominal_value=1
  PS-Simulink Converter2 : nesl_utility/PS-Simulink Converter  PhysicalDomain=network_engine_domain  SubClassName=ps_output  LeftPortType=input  RightPortType=output  PseudoPeriodic=off  Frequencies=[]  VectorFormat=1-D array  Unit=1  AffineConversion=off
  "Qc - Qj " : Subsystem
  "Qc - Qj1 " : fl_lib/Thermal/Thermal Sources/Controlled Heat Flow Rate Source
  Qh  + Qj : fl_lib/Thermal/Thermal Sources/Controlled Heat Flow Rate Source
  "Qh + Qj " : Subsystem
  ReC : fl_lib/Electrical/Electrical Elements/Resistor  R=ReC Ohm  i_specify=off  i_priority=None  i=0 A  i_nominal_specify=off  i_nominal_unit=A  i_nominal_value=1  v_specify=off  v_priority=None  v=0 V  v_nominal_specify=off  v_nominal_unit=V  v_nominal_value=1
  Rth : fl_lib/Thermal/Thermal Elements/Thermal Resistance  resistance=Rth K/W  T_specify=off  T_priority=None  T=0 K  T_nominal_specify=off  T_nominal_unit=K  T_nominal_value=1  Q_specify=off  Q_priority=None  Q=0 W  Q_nominal_specify=off  Q_nominal_unit=W  Q_nominal_value=1
  Saturation : Saturate  UpperLimit=inf  LowerLimit=-inf
  Scope : Scope
  Scope2 : Scope
  Simulink-PS Converter : nesl_utility/Simulink-PS Converter  PhysicalDomain=network_engine_domain  SubClassName=ps_input  LeftPortType=input  RightPortType=output  PseudoPeriodic=off  Frequencies=[]  NoiseDistribution=none  NoiseParameters=[]  Unit=1  AffineConversion=off  FilteringAndDerivatives=provide  SimscapeFilterOrder=1  InputFilterTimeConstant=0.001  UdotUserProvided=0
  Subsystem : Subsystem
  Tc : Scope
  Thermal Reference1 : fl_lib/Thermal/Thermal Elements/Thermal Reference
  Thermal Reference2 : fl_lib/Thermal/Thermal Elements/Thermal Reference
  dT1 : Scope
  TC : PMIOPort  Side=Right
  V+ : PMIOPort  Port=2  Side=Left
  V- : PMIOPort  Port=3  Side=Left
  TH : PMIOPort  Port=4  Side=Right
  wires:
  Gain2/1 -> Add/1
  Add/1 -> Simulink-PS Converter/1
  Constant/1 -> Gain2/1
  Gain1/1 -> Add/2
  Gain/1 -> Gain1/1
  Subsystem/3(dT) -> dT1/1, Gain/1
  Saturation/1 -> 0.5 x I^2 x ReC/1(In1), Alpha x I x Th/2(I)
  Subsystem/2(Th) -> Alpha x I x Th/1(T), Scope2/1
  Alpha x I x Th/2(Out2) -> "Qh + Qj "/1(In1)
  Alpha x I x Tc/1 -> "Qc - Qj "/1(In1)
  Alpha x I x Th/1(Out1) -> Alpha x I x Tc/2
  Subsystem/1(Tc) -> Alpha x I x Tc/1, Tc/1
  0.5 x I^2 x ReC/1(Out1) -> "Qh + Qj "/2(In2), "Qc - Qj "/2(In2)
  PS-Simulink Converter2/1 -> Saturation/1, Scope/1
  connections:
  Rth/LConn1 -- TC/RConn1 -- Mc1/LConn1 -- Subsystem/LConn1 -- "Qc - Qj1 "/RConn2
  "Qh + Qj "/RConn1 -- Qh  + Qj/RConn1
  "Qc - Qj1 "/RConn1 -- "Qc - Qj "/RConn1
  Electrical Reference1/LConn1 -- V-/RConn1 -- Current Sensor/RConn2
  Controlled Voltage Source/LConn1 -- V+/RConn1
  PS-Simulink Converter2/LConn1 -- Current Sensor/RConn1
  Controlled Voltage Source/RConn2 -- ReC/LConn1
  Simulink-PS Converter/RConn1 -- Controlled Voltage Source/RConn1
  TH/RConn1 -- Subsystem/LConn2 -- Qh  + Qj/LConn1 -- Rth/RConn1 -- Mh/LConn1
  Thermal Reference2/LConn1 -- Qh  + Qj/RConn2
  Thermal Reference1/LConn1 -- "Qc - Qj1 "/LConn1
  Current Sensor/LConn1 -- ReC/RConn1

== system A1_MIM0_DigiTwin_4cm_JG_BM_2017b/Subsystem5/Subsystem1 ==
  PS-Simulink Converter7 : nesl_utility/PS-Simulink Converter  PhysicalDomain=network_engine_domain  SubClassName=ps_output  LeftPortType=input  RightPortType=output  PseudoPeriodic=off  Frequencies=[]  VectorFormat=1-D array  Unit=1  AffineConversion=off
  Temperature Sensor1 : fl_lib/Thermal/Thermal Sensors/Temperature Sensor
  Thermal Reference2 : fl_lib/Thermal/Thermal Elements/Thermal Reference
  Conn1 : PMIOPort  Side=Left
  Out1 : Outport  VectorParamsAs1DForOutWhenUnconnected=off
  wires:
  PS-Simulink Converter7/1 -> Out1/1
  connections:
  Temperature Sensor1/LConn1 -- Conn1/RConn1
  PS-Simulink Converter7/LConn1 -- Temperature Sensor1/RConn2
  Thermal Reference2/LConn1 -- Temperature Sensor1/RConn1

== system A1_MIM0_DigiTwin_4cm_JG_BM_2017b/Subsystem1/P2/0.5 x I^2 x ReC ==
  In1 : Inport
  Constant1 : Constant  Value=0.5*ReC
  Product1 : Product  Inputs=3
  Out1 : Outport  VectorParamsAs1DForOutWhenUnconnected=off
  wires:
  Constant1/1 -> Product1/1
  Product1/1 -> Out1/1
  In1/1 -> Product1/3, Product1/2

== system A1_MIM0_DigiTwin_4cm_JG_BM_2017b/Subsystem1/P2/Alpha x I x Th ==
  note: Alpha x I
  T : Inport
  I : Inport  Port=2
  Constant : Constant  Value=am
  Product : Product
  Product2 : Product
  Out1 : Outport  VectorParamsAs1DForOutWhenUnconnected=off
  Out2 : Outport  Port=2  VectorParamsAs1DForOutWhenUnconnected=off
  wires:
  T/1 -> Product2/1
  Constant/1 -> Product/1
  I/1 -> Product/2
  Product2/1 -> Out2/1
  Product/1 -> Out1/1, Product2/2

== system A1_MIM0_DigiTwin_4cm_JG_BM_2017b/Subsystem1/P2/Qc - Qj  ==
  In1 : Inport
  In2 : Inport  Port=2
  Add1 : Sum  Inputs=+-
  Scope5 : Scope
  Simulink-PS Converter1 : nesl_utility/Simulink-PS Converter  PhysicalDomain=network_engine_domain  SubClassName=ps_input  LeftPortType=input  RightPortType=output  PseudoPeriodic=off  Frequencies=[]  NoiseDistribution=none  NoiseParameters=[]  Unit=1  AffineConversion=off  FilteringAndDerivatives=provide  SimscapeFilterOrder=1  InputFilterTimeConstant=0.001  UdotUserProvided=0
  Conn1 : PMIOPort  Side=Right
  wires:
  Add1/1 -> Scope5/1, Simulink-PS Converter1/1
  In1/1 -> Add1/1
  In2/1 -> Add1/2
  connections:
  Conn1/RConn1 -- Simulink-PS Converter1/RConn1

== system A1_MIM0_DigiTwin_4cm_JG_BM_2017b/Subsystem1/P2/Qh + Qj  ==
  In1 : Inport
  In2 : Inport  Port=2
  Add : Sum
  Scope4 : Scope
  Simulink-PS Converter2 : nesl_utility/Simulink-PS Converter  PhysicalDomain=network_engine_domain  SubClassName=ps_input  LeftPortType=input  RightPortType=output  PseudoPeriodic=off  Frequencies=[]  NoiseDistribution=none  NoiseParameters=[]  Unit=1  AffineConversion=off  FilteringAndDerivatives=provide  SimscapeFilterOrder=1  InputFilterTimeConstant=0.001  UdotUserProvided=0
  Conn1 : PMIOPort  Side=Right
  wires:
  Add/1 -> Scope4/1, Simulink-PS Converter2/1
  In2/1 -> Add/2
  In1/1 -> Add/1
  connections:
  Simulink-PS Converter2/RConn1 -- Conn1/RConn1

== system A1_MIM0_DigiTwin_4cm_JG_BM_2017b/Subsystem1/P2/Subsystem ==
  PS-Simulink Converter : nesl_utility/PS-Simulink Converter  PhysicalDomain=network_engine_domain  SubClassName=ps_output  LeftPortType=input  RightPortType=output  PseudoPeriodic=off  Frequencies=[]  VectorFormat=1-D array  Unit=1  AffineConversion=off
  PS-Simulink Converter1 : nesl_utility/PS-Simulink Converter  PhysicalDomain=network_engine_domain  SubClassName=ps_output  LeftPortType=input  RightPortType=output  PseudoPeriodic=off  Frequencies=[]  VectorFormat=1-D array  Unit=1  AffineConversion=off
  Subtract1 : Sum  Inputs=-+
  Temperature Sensor : fl_lib/Thermal/Thermal Sensors/Temperature Sensor
  Temperature Sensor1 : fl_lib/Thermal/Thermal Sensors/Temperature Sensor
  Thermal Reference1 : fl_lib/Thermal/Thermal Elements/Thermal Reference
  Thermal Reference4 : fl_lib/Thermal/Thermal Elements/Thermal Reference
  Tcold : PMIOPort  Side=Left
  Thot : PMIOPort  Port=2  Side=Left
  Tc : Outport  VectorParamsAs1DForOutWhenUnconnected=off
  Th : Outport  Port=2  VectorParamsAs1DForOutWhenUnconnected=off
  dT : Outport  Port=3  VectorParamsAs1DForOutWhenUnconnected=off
  wires:
  PS-Simulink Converter1/1 -> Th/1, Subtract1/2
  Subtract1/1 -> dT/1
  PS-Simulink Converter/1 -> Subtract1/1, Tc/1
  connections:
  Thot/RConn1 -- Temperature Sensor1/LConn1
  Tcold/RConn1 -- Temperature Sensor/LConn1
  PS-Simulink Converter/LConn1 -- Temperature Sensor/RConn2
  Thermal Reference4/LConn1 -- Temperature Sensor/RConn1
  PS-Simulink Converter1/LConn1 -- Temperature Sensor1/RConn2
  Thermal Reference1/LConn1 -- Temperature Sensor1/RConn1

== system A1_MIM0_DigiTwin_4cm_JG_BM_2017b/Subsystem5/P2/0.5 x I^2 x ReC ==
  In1 : Inport
  Constant1 : Constant  Value=0.5*ReC
  Product1 : Product  Inputs=3
  Out1 : Outport  VectorParamsAs1DForOutWhenUnconnected=off
  wires:
  In1/1 -> Product1/2, Product1/3
  Product1/1 -> Out1/1
  Constant1/1 -> Product1/1

== system A1_MIM0_DigiTwin_4cm_JG_BM_2017b/Subsystem5/P2/Alpha x I x Th ==
  note: Alpha x I
  T : Inport
  I : Inport  Port=2
  Constant : Constant  Value=am
  Product : Product
  Product2 : Product
  Out1 : Outport  VectorParamsAs1DForOutWhenUnconnected=off
  Out2 : Outport  Port=2  VectorParamsAs1DForOutWhenUnconnected=off
  wires:
  Product/1 -> Product2/2, Out1/1
  Product2/1 -> Out2/1
  I/1 -> Product/2
  Constant/1 -> Product/1
  T/1 -> Product2/1

== system A1_MIM0_DigiTwin_4cm_JG_BM_2017b/Subsystem5/P2/Qc - Qj  ==
  In1 : Inport
  In2 : Inport  Port=2
  Add1 : Sum  Inputs=+-
  Scope5 : Scope
  Simulink-PS Converter1 : nesl_utility/Simulink-PS Converter  PhysicalDomain=network_engine_domain  SubClassName=ps_input  LeftPortType=input  RightPortType=output  PseudoPeriodic=off  Frequencies=[]  NoiseDistribution=none  NoiseParameters=[]  Unit=1  AffineConversion=off  FilteringAndDerivatives=provide  SimscapeFilterOrder=1  InputFilterTimeConstant=0.001  UdotUserProvided=0
  Conn1 : PMIOPort  Side=Right
  wires:
  In2/1 -> Add1/2
  In1/1 -> Add1/1
  Add1/1 -> Simulink-PS Converter1/1, Scope5/1
  connections:
  Conn1/RConn1 -- Simulink-PS Converter1/RConn1

== system A1_MIM0_DigiTwin_4cm_JG_BM_2017b/Subsystem5/P2/Qh + Qj  ==
  In1 : Inport
  In2 : Inport  Port=2
  Add : Sum
  Scope4 : Scope
  Simulink-PS Converter2 : nesl_utility/Simulink-PS Converter  PhysicalDomain=network_engine_domain  SubClassName=ps_input  LeftPortType=input  RightPortType=output  PseudoPeriodic=off  Frequencies=[]  NoiseDistribution=none  NoiseParameters=[]  Unit=1  AffineConversion=off  FilteringAndDerivatives=provide  SimscapeFilterOrder=1  InputFilterTimeConstant=0.001  UdotUserProvided=0
  Conn1 : PMIOPort  Side=Right
  wires:
  In1/1 -> Add/1
  In2/1 -> Add/2
  Add/1 -> Simulink-PS Converter2/1, Scope4/1
  connections:
  Simulink-PS Converter2/RConn1 -- Conn1/RConn1

== system A1_MIM0_DigiTwin_4cm_JG_BM_2017b/Subsystem5/P2/Subsystem ==
  PS-Simulink Converter : nesl_utility/PS-Simulink Converter  PhysicalDomain=network_engine_domain  SubClassName=ps_output  LeftPortType=input  RightPortType=output  PseudoPeriodic=off  Frequencies=[]  VectorFormat=1-D array  Unit=1  AffineConversion=off
  PS-Simulink Converter1 : nesl_utility/PS-Simulink Converter  PhysicalDomain=network_engine_domain  SubClassName=ps_output  LeftPortType=input  RightPortType=output  PseudoPeriodic=off  Frequencies=[]  VectorFormat=1-D array  Unit=1  AffineConversion=off
  Subtract1 : Sum  Inputs=-+
  Temperature Sensor : fl_lib/Thermal/Thermal Sensors/Temperature Sensor
  Temperature Sensor1 : fl_lib/Thermal/Thermal Sensors/Temperature Sensor
  Thermal Reference1 : fl_lib/Thermal/Thermal Elements/Thermal Reference
  Thermal Reference4 : fl_lib/Thermal/Thermal Elements/Thermal Reference
  Tcold : PMIOPort  Side=Left
  Thot : PMIOPort  Port=2  Side=Left
  Tc : Outport  VectorParamsAs1DForOutWhenUnconnected=off
  Th : Outport  Port=2  VectorParamsAs1DForOutWhenUnconnected=off
  dT : Outport  Port=3  VectorParamsAs1DForOutWhenUnconnected=off
  wires:
  PS-Simulink Converter/1 -> Tc/1, Subtract1/1
  Subtract1/1 -> dT/1
  PS-Simulink Converter1/1 -> Subtract1/2, Th/1
  connections:
  Thermal Reference1/LConn1 -- Temperature Sensor1/RConn1
  PS-Simulink Converter1/LConn1 -- Temperature Sensor1/RConn2
  Thermal Reference4/LConn1 -- Temperature Sensor/RConn1
  PS-Simulink Converter/LConn1 -- Temperature Sensor/RConn2
  Tcold/RConn1 -- Temperature Sensor/LConn1
  Thot/RConn1 -- Temperature Sensor1/LConn1
